simulink model "project1_bonus_rlc_circuit"  (R2021b)
settings: Solver=ode23tb  StartTime=0.0  StopTime=0.2  RelTol=1e-3
libraries: spsSeriesRLCBranchLib x12, spsGroundLib x6, spsVoltageMeasurementLib x4, spsCurrentMeasurementLib x3, spsIdealSwitchLib x3, spsStairGeneratorLib x1, spsThreePhaseProgrammableVoltageSourceLib x1, spspowerguiLib x1
settings Model: Creator=naeem  LastModifiedBy=nolo7
settings SolverCC: AlgebraicLoopSolver=TrustRegion
settings DebuggingCC: SFMachineParentedDataDiag=warning

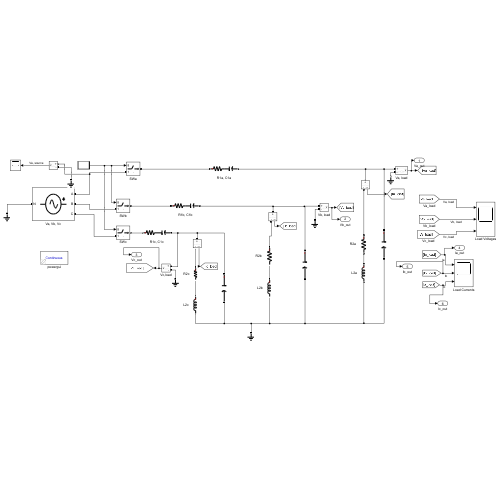
[thumbnail: Simulink's stored preview of the top-level diagram]
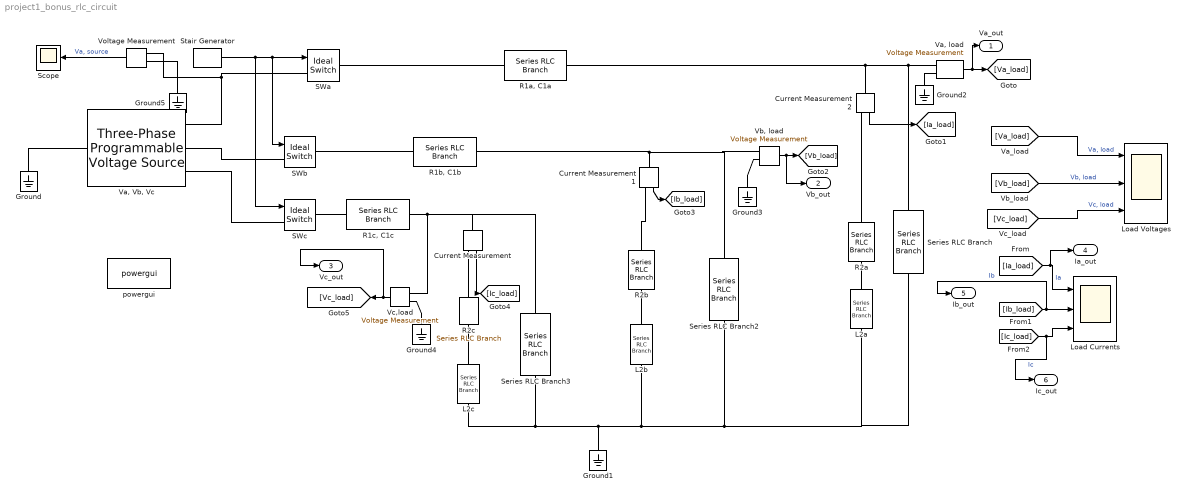
== system project1_bonus_rlc_circuit ==
  Current Measurement : spsCurrentMeasurementLib/Current Measurement  PhasorSimulation=off  OutputType=Complex  PSBequivalent=0
  Current Measurement1 : spsCurrentMeasurementLib/Current Measurement  PhasorSimulation=off  OutputType=Complex  PSBequivalent=0
  Current Measurement2 : spsCurrentMeasurementLib/Current Measurement  PhasorSimulation=off  OutputType=Complex  PSBequivalent=0
  Ground{,1..5} (6 alike) : spsGroundLib/Ground  LConnTagsString=a
  L2a : spsSeriesRLCBranchLib/Series RLC Branch  LConnTagsString=__new0  RConnTagsString=__new0  BranchType=L  Resistance=1  Inductance=5e-3  SetiL0=off  InitialCurrent=0  Capacitance=1e-6  Setx0=off  InitialVoltage=0  Measurements=None
  L2b : spsSeriesRLCBranchLib/Series RLC Branch  LConnTagsString=__new0  RConnTagsString=__new0  BranchType=L  Resistance=1  Inductance=10e-3  SetiL0=on  InitialCurrent=0  Capacitance=1e-6  Setx0=off  InitialVoltage=0  Measurements=None
  L2c : spsSeriesRLCBranchLib/Series RLC Branch  LConnTagsString=__new0  RConnTagsString=__new0  BranchType=L  Resistance=1  Inductance=15e-3  SetiL0=on  InitialCurrent=0  Capacitance=1e-6  Setx0=off  InitialVoltage=0  Measurements=None
  Load Currents : Scope  NumInputPorts=3
  Load Voltages : Scope  NumInputPorts=3
  "R1a, C1a" : spsSeriesRLCBranchLib/Series RLC Branch  LConnTagsString=__new0  RConnTagsString=__new0  BranchType=RC  Resistance=0.1  Inductance=0.1  SetiL0=off  InitialCurrent=0  Capacitance=10e-6  Setx0=on  InitialVoltage=0  Measurements=None
  "R1b, C1b" : spsSeriesRLCBranchLib/Series RLC Branch  LConnTagsString=__new0  RConnTagsString=__new0  BranchType=RC  Resistance=0.1  Inductance=0.1  SetiL0=off  InitialCurrent=0  Capacitance=10e-6  Setx0=on  InitialVoltage=0  Measurements=None
  "R1c, C1c" : spsSeriesRLCBranchLib/Series RLC Branch  LConnTagsString=__new0  RConnTagsString=__new0  BranchType=RC  Resistance=0.1  Inductance=0.1  SetiL0=off  InitialCurrent=0  Capacitance=10e-6  Setx0=on  InitialVoltage=0  Measurements=None
  R2a : spsSeriesRLCBranchLib/Series RLC Branch  LConnTagsString=__new0  RConnTagsString=__new0  BranchType=R  Resistance=5  Inductance=1e-3  SetiL0=off  InitialCurrent=0  Capacitance=1e-6  Setx0=off  InitialVoltage=0  Measurements=None
  R2b : spsSeriesRLCBranchLib/Series RLC Branch  LConnTagsString=__new0  RConnTagsString=__new0  BranchType=R  Resistance=2.5  Inductance=1e-3  SetiL0=off  InitialCurrent=0  Capacitance=1e-6  Setx0=off  InitialVoltage=0  Measurements=None
  R2c : spsSeriesRLCBranchLib/Series RLC Branch  LConnTagsString=__new0  RConnTagsString=__new0  BranchType=R  Resistance=10  Inductance=1e-3  SetiL0=off  InitialCurrent=0  Capacitance=1e-6  Setx0=off  InitialVoltage=0  Measurements=None
  SWa : spsIdealSwitchLib/Ideal Switch  Ron=0.01  Lon=1e-9  IC=1  Rs=inf  Cs=0  Measurements=off
      settings: AttributesFormatString=\n
  "SWb " : spsIdealSwitchLib/Ideal Switch  Ron=0.01  Lon=1e-9  IC=1  Rs=inf  Cs=0  Measurements=off
      settings: AttributesFormatString=\n
  SWc : spsIdealSwitchLib/Ideal Switch  Ron=0.01  Lon=1e-9  IC=1  Rs=inf  Cs=0  Measurements=off
      settings: AttributesFormatString=\n
  Scope : Scope
  Series RLC Branch : spsSeriesRLCBranchLib/Series RLC Branch  LConnTagsString=__new0  RConnTagsString=__new0  BranchType=C  Resistance=1  Inductance=1e-3  SetiL0=off  InitialCurrent=0  Capacitance=50e-6  Setx0=on  InitialVoltage=0  Measurements=None
  Series RLC Branch2 : spsSeriesRLCBranchLib/Series RLC Branch  LConnTagsString=__new0  RConnTagsString=__new0  BranchType=C  Resistance=1  Inductance=1e-3  SetiL0=off  InitialCurrent=0  Capacitance=50e-6  Setx0=on  InitialVoltage=0  Measurements=None
  Series RLC Branch3 : spsSeriesRLCBranchLib/Series RLC Branch  LConnTagsString=__new0  RConnTagsString=__new0  BranchType=C  Resistance=1  Inductance=1e-3  SetiL0=off  InitialCurrent=0  Capacitance=50e-6  Setx0=on  InitialVoltage=0  Measurements=None
  Stair Generator : spsStairGeneratorLib/Stair Generator  t="[0 3/60  8.25/60 ]"  e=[1 0 1]  Ts=0
  "Va, Vb, Vc" : spsThreePhaseProgrammableVoltageSourceLib/Three-Phase Programmable Voltage Source  PositiveSequence=[120.0 0 60]  VariationEntity=None  VariationType=Table of time-amplitude pairs  VariationTypeAlt=Step  VariationStep=0.5  VariationRate=10  VariationMagnitude=0.3  VariationFrequency=2  VariationTiming=[1 2]  VariationPhaseA=off  Amplitudes=[1 0.8 1.2 1.0]  TimeValues=[0 0.1 0.15 0.2]  HarmonicGeneration=off  HarmonicA=[3 0.2 -25 0]  HarmonicB=[2 0.15 35 2]  Timing="[0.05  3]"  BusType=swing  Pref=0  Qref=0  Qmin=-inf  Qmax=inf
  "Va, load" : spsVoltageMeasurementLib/Voltage Measurement  PhasorSimulation=off  OutputType=Complex  PSBequivalent=0
  "Vb, load" : spsVoltageMeasurementLib/Voltage Measurement  PhasorSimulation=off  OutputType=Complex  PSBequivalent=0
  Vc,load : spsVoltageMeasurementLib/Voltage Measurement  PhasorSimulation=off  OutputType=Complex  PSBequivalent=0
  Voltage Measurement : spsVoltageMeasurementLib/Voltage Measurement  PhasorSimulation=off  OutputType=Complex  PSBequivalent=0
  powergui : spspowerguiLib/powergui  Priority=1  SimulationMode=Continuous  SampleTime=50e-6  frequency=60  Iterations=50  frequencyindice=60  Pbase=100e6  ErrMax=1e-4  UnitsV=kV  UnitsW=MW  buscounter=0  FunctionMessages=off  echomessages=off  EnableUseOfTLC=off  CurrentSourceSwitches=off  DisableSnubberDevices=off  DisableRonSwitches=off  DisableVfSwitches=off  DisplayEquations=off  AutomaticDiscreteSolvers=off  SolverType=Tustin/Backward Euler (TBE)  Interpol=off  ExternalGateDelay=off  methode=off  Ts=100  x0status=zero  SPID=on  SwTol=0  HookPort=off  NonlinearTolerance=1e-4  nMaxIteration=100  ContinueOnMaxIteration=off  RestoreLinks=warning  ResistiveCurrentMeasurement=off  Frange=[0:2:500]  Ylog=off  Xlog=on  ShowGrid=off  save=off  variable=ZData  structure=0  ZoomFFT=off  StartTime=0.0  cycles=1  DisplayStyle=1  fundamental=60  FreqAxis=off  MaxFrequency=1000  frequencyindicesteady=1  RmsSteady=1  display=off
  Va_out : Outport
  Vb_out : Outport  Port=2
  Vc_out : Outport  Port=3
  Ia_out : Outport  Port=4
  Ib_out : Outport  Port=5
  Ic_out : Outport  Port=6
  wires:
  "Va, load"/1 -> Va_out/1, [Va_load]
  [Va_load] -> Load Voltages/1  "Va, load"
  Current Measurement2/1 -> [Ia_load]
  [Ia_load] -> Ia_out/1, Load Currents/1  "Ia"
  [Vb_load] -> Load Voltages/2  "Vb, load"
  "Vb, load"/1 -> Vb_out/1, [Vb_load]
  Current Measurement1/1 -> [Ib_load]
  [Ib_load] -> Ib_out/1, Load Currents/2  "Ib"
  Current Measurement/1 -> [Ic_load]
  Vc,load/1 -> Vc_out/1, [Vc_load]
  [Vc_load] -> Load Voltages/3  "Vc, load"
  [Ic_load] -> Ic_out/1, Load Currents/3  "Ic"
  Stair Generator/1 -> SWc/1, "SWb "/1, SWa/1
  Voltage Measurement/1 -> Scope/1  "Va, source"
  connections:
  Ground/LConn1 -- "Va, Vb, Vc"/LConn1
  "Va, load"/LConn1 -- Current Measurement2/LConn1 -- "R1a, C1a"/RConn1 -- Series RLC Branch/LConn1
  L2c/RConn1 -- Series RLC Branch/RConn1 -- L2a/RConn1 -- Series RLC Branch2/RConn1 -- L2b/RConn1 -- Ground1/LConn1 -- Series RLC Branch3/RConn1
  SWa/LConn1 -- "Va, Vb, Vc"/RConn1 -- Voltage Measurement/LConn1
  SWa/RConn1 -- "R1a, C1a"/LConn1
  "Va, Vb, Vc"/RConn2 -- "SWb "/LConn1
  "R1b, C1b"/LConn1 -- "SWb "/RConn1
  SWc/RConn1 -- "R1c, C1c"/LConn1
  SWc/LConn1 -- "Va, Vb, Vc"/RConn3
  L2a/LConn1 -- R2a/RConn1
  Current Measurement2/RConn1 -- R2a/LConn1
  Ground2/LConn1 -- "Va, load"/LConn2
  Current Measurement1/RConn1 -- R2b/LConn1
  Current Measurement1/LConn1 -- "Vb, load"/LConn1 -- Series RLC Branch2/LConn1 -- "R1b, C1b"/RConn1
  L2b/LConn1 -- R2b/RConn1
  Ground3/LConn1 -- "Vb, load"/LConn2
  "R1c, C1c"/RConn1 -- Series RLC Branch3/LConn1 -- Current Measurement/LConn1 -- Vc,load/LConn1
  Current Measurement/RConn1 -- R2c/LConn1
  R2c/RConn1 -- L2c/LConn1
  Ground4/LConn1 -- Vc,load/LConn2
  Ground5/LConn1 -- Voltage Measurement/LConn2
